simulink model "Lab1bPartA1"  (R2023b)
settings: Solver=VariableStepAuto  StartTime=0.0  StopTime=30  RelTol=1e-3
settings Model: Creator=tanvi  LastModifiedBy=tanvi

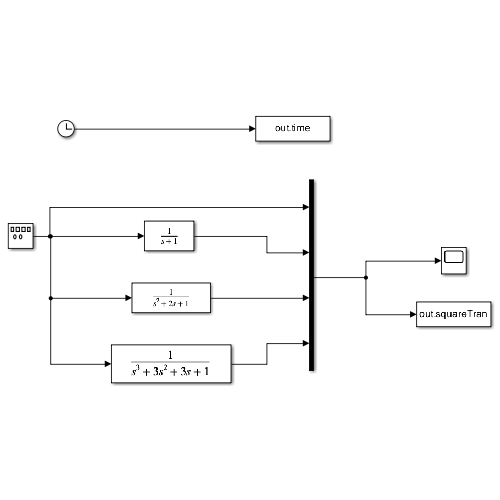
[thumbnail: Simulink's stored preview of the top-level diagram]
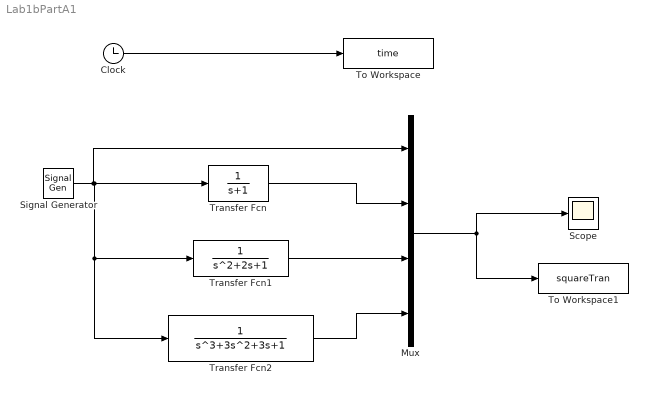
== system Lab1bPartA1 ==
  Clock : Clock
      settings: Decimation=100
  Mux : Mux
  Scope : Scope
  Signal Generator : SignalGenerator  WaveForm=square  Frequency=0.05
  To Workspace : ToWorkspace  VariableName=time  SampleTime=-1
  To Workspace1 : ToWorkspace  VariableName=squareTran  SampleTime=-1
  Transfer Fcn : TransferFcn  Denominator=[1 1]
  Transfer Fcn1 : TransferFcn
  Transfer Fcn2 : TransferFcn  Denominator=[1 3 3 1]
  wires:
  Signal Generator/1 -> Transfer Fcn2/1, Transfer Fcn1/1, Transfer Fcn/1, Mux/1
  Clock/1 -> To Workspace/1
  Mux/1 -> To Workspace1/1, Scope/1
  Transfer Fcn/1 -> Mux/2
  Transfer Fcn2/1 -> Mux/4
  Transfer Fcn1/1 -> Mux/3
